simulink model "DC_Motor_Using_TransfertFunction"  (R2018a)
settings: Solver=VariableStepAuto  StartTime=0.0  StopTime=10.0  RelTol=1e-3
libraries: simulink x1
settings Model: Creator=Jayef  LastModifiedBy=Jayef

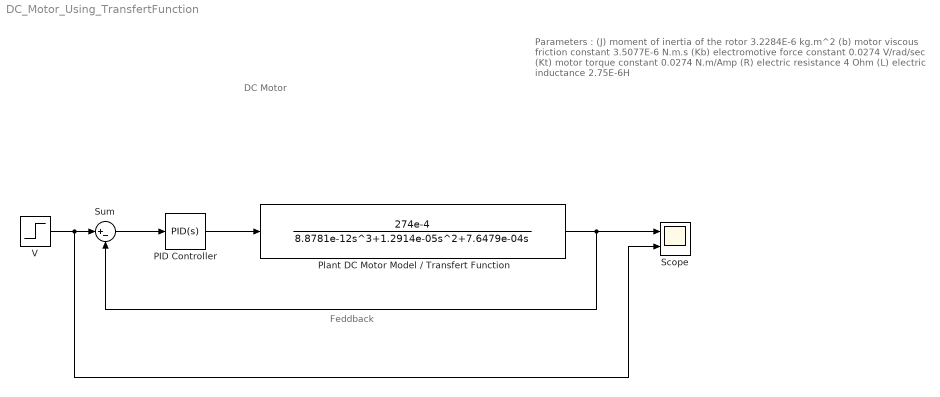
== system DC_Motor_Using_TransfertFunction ==
  note: Feddback
  note: DC Motor
  note: Parameters :
      | (J) moment of inertia of the rotor 3.2284E-6 kg.m^2
      | (b) motor viscous friction constant 3.5077E-6 N.m.s
      | (Kb) electromotive force constant 0.0274 V/rad/sec
      | (Kt) motor torque constant 0.0274 N.m/Amp
      | (R) electric resistance 4 Ohm
      | (L) electric inductance 2.75E-6H
  PID Controller : simulink/Continuous/PID Controller  Controller=PID  TimeDomain=Continuous-time  SampleTime=-1  IntegratorMethod=Forward Euler  FilterMethod=Forward Euler  Form=Parallel  UseFilter=on  ControllerParametersSource=internal  P=0.691453365618904  I=3.09706546267757  D=0.00903847659465251  N=37.4582307494942  InitialConditionSource=internal  InitialConditionForIntegrator=0  InitialConditionForFilter=0  ExternalReset=none  LimitOutput=off  UpperSaturationLimit=inf  LowerSaturationLimit=-inf  LinearizeAsGain=on  AntiWindupMode=none  Kb=1  TrackingMode=off  Kt=1  PParamMin=[]  PParamMax=[]  IParamMin=[]  IParamMax=[]  DParamMin=[]  DParamMax=[]  NParamMin=[]  NParamMax=[]  KbParamMin=[]  KbParamMax=[]  KtParamMin=[]  KtParamMax=[]  POutMin=[]  POutMax=[]  IOutMin=[]  IOutMax=[]  DOutMin=[]  DOutMax=[]  NOutMin=[]  NOutMax=[]  KbOutMin=[]  KbOutMax=[]  KtOutMin=[]  KtOutMax=[]  IntegratorOutMin=[]  IntegratorOutMax=[]  FilterOutMin=[]  FilterOutMax=[]  SumOutMin=[]  SumOutMax=[]  SumI1OutMin=[]  SumI1OutMax=[]  SumI2OutMin=[]  SumI2OutMax=[]  SumI3OutMin=[]  SumI3OutMax=[]  SumDOutMin=[]  SumDOutMax=[]  SaturationOutMin=[]  SaturationOutMax=[]  IntegratorContinuousStateAttributes=''  IntegratorStateMustResolveToSignalObject=off  IntegratorRTWStateStorageClass=Auto  FilterContinuousStateAttributes=''  FilterStateMustResolveToSignalObject=off  FilterRTWStateStorageClass=Auto  DifferentiatorICPrevScaledInput=0  DifferentiatorOutMin=[]  DifferentiatorOutMax=[]  FilterDiffOutCoefMin=[]  FilterDiffOutCoefMax=[]  SumDenOutMin=[]  SumDenOutMax=[]  SumNumOutMin=[]  SumNumOutMax=[]  ReciprocalOutMin=[]  ReciprocalOutMax=[]  DivideOutMin=[]  DivideOutMax=[]  TunerSelectOption=Transfer Function Based (PID Tuner App)
  Plant DC Motor Model / Transfert Function : TransferFcn  Numerator=[274e-4]  Denominator=[8.8781e-12 1.2914e-05 7.6479e-04 0]
  Scope : Scope  NumInputPorts=2
  Sum : Sum  Inputs=|+-
  V : Step  SampleTime=0
  wires:
  Plant DC Motor Model / Transfert Function/1 -> Sum/2, Scope/1
  V/1 -> Scope/2, Sum/1
  Sum/1 -> PID Controller/1
  PID Controller/1 -> Plant DC Motor Model / Transfert Function/1
